simulink subsystem "Alfa_e_Mach"  (R2024b)
settings: Solver=VariableStepAuto  StartTime=0.0  StopTime=10.0  RelTol=1e-3
libraries: aerolibasang x3
settings Model: Creator=joedo  LastModifiedBy=joedo

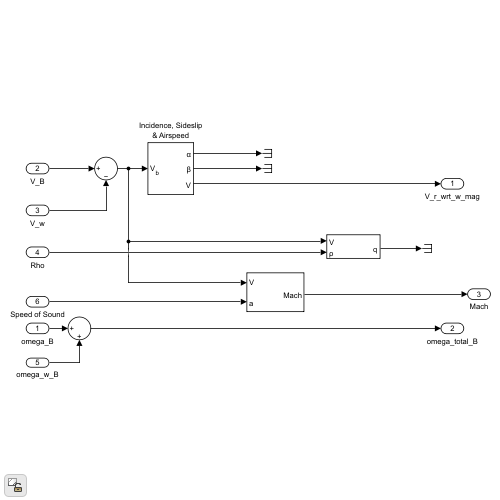
[thumbnail: Simulink's stored preview of the top-level diagram]
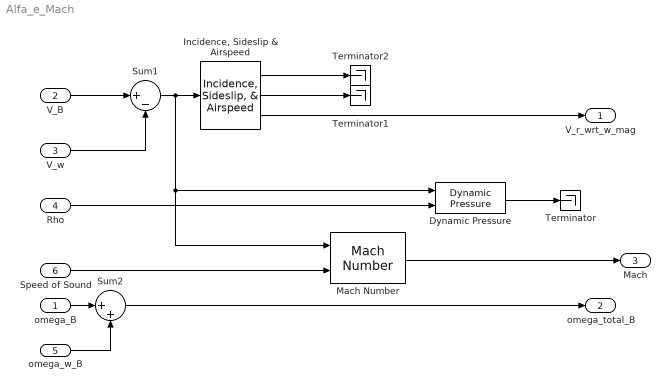
== system Alfa_e_Mach ==
  omega_B : Inport
  V_B : Inport  Port=2
  V_w : Inport  Port=3
  Rho : Inport  Port=4
  omega_w_B : Inport  Port=5
  Speed of Sound : Inport  Port=6  Unit=m/s
  Dynamic Pressure : aerolibasang/Dynamic Pressure
  "Incidence, Sideslip & Airspeed" : aerolibasang/Incidence, Sideslip, & Airspeed
  Mach Number : aerolibasang/Mach Number
  Sum1 : Sum  Inputs=|+-  InputSameDT=on  SaturateOnIntegerOverflow=on  OutDataTypeStr=Inherit: Same as first input
  Sum2 : Sum  Inputs=|++  InputSameDT=on  SaturateOnIntegerOverflow=on  OutDataTypeStr=Inherit: Same as first input
  Terminator : Terminator
  Terminator1 : Terminator
  Terminator2 : Terminator
  V_r_wrt_w_mag : Outport  VectorParamsAs1DForOutWhenUnconnected=off
  omega_total_B : Outport  Port=2  VectorParamsAs1DForOutWhenUnconnected=off
  Mach : Outport  Port=3  VectorParamsAs1DForOutWhenUnconnected=off
  wires:
  V_w/1 -> Sum1/2
  Rho/1 -> Dynamic Pressure/2
  Dynamic Pressure/1 -> Terminator/1
  "Incidence, Sideslip & Airspeed"/3 -> V_r_wrt_w_mag/1
  omega_B/1 -> Sum2/1
  omega_w_B/1 -> Sum2/2
  Sum2/1 -> omega_total_B/1
  V_B/1 -> Sum1/1
  Mach Number/1 -> Mach/1
  Sum1/1 -> Mach Number/1, Dynamic Pressure/1, "Incidence, Sideslip & Airspeed"/1
  Speed of Sound/1 -> Mach Number/2
  "Incidence, Sideslip & Airspeed"/2 -> Terminator1/1
  "Incidence, Sideslip & Airspeed"/1 -> Terminator2/1
